simulink library "lib_wheel_nodiv"  (Simulink 7.7)
settings: Solver=ode45  SolverMode=SingleTasking  StartTime=0.0  StopTime=10.0  RelTol=1e-3
undefined symbols (not defined in the file): Fc_table_x, Fc_table_y, I, R, T_veh, use_division, w0, w_max
settings Model: Creator=yt59680  LastModifiedBy=lfeng

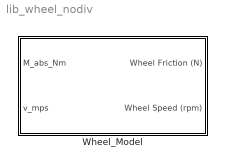
== system lib_wheel_nodiv ==
  Wheel_Model : Subsystem  TreatAsAtomicUnit=on

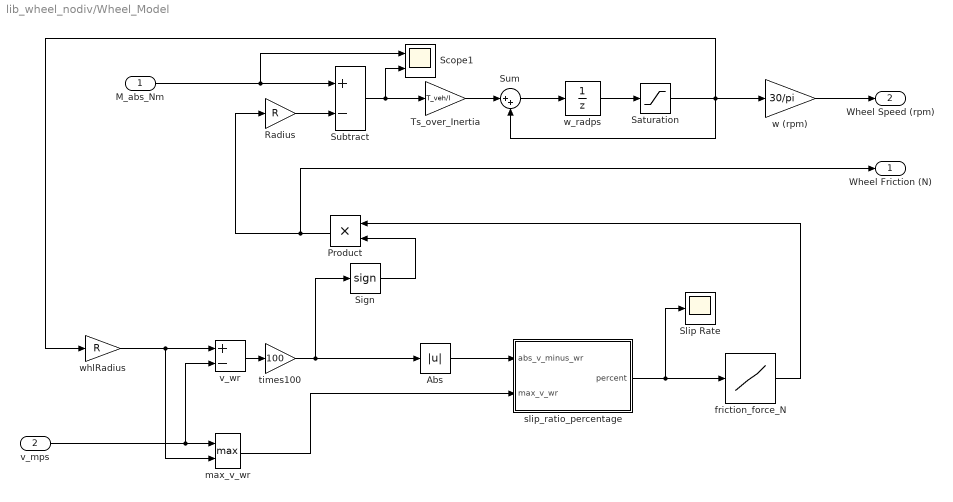
== system lib_wheel_nodiv/Wheel_Model ==
  M_abs_Nm : Inport
  v_mps : Inport  Port=2
  Abs : Abs
  Product : Product  RndMeth=Zero
  Radius : Gain  Gain=R
  Saturation : Saturate  UpperLimit=w_max  LowerLimit=0
  Scope1 : Scope  NumInputPorts=2
      settings: YMin=-5~-5  YMax=5~5  SaveName=ScopeData7
  Sign : Signum
  Slip Rate : Scope
      settings: SaveName=ScopeData8
  Subtract : Sum  Inputs=+-
  Sum : Sum  Inputs=|++
  Ts_over_Inertia : Gain  Gain=T_veh/I
  friction_force_N : Lookup  InputValues=Fc_table_x  Table=Fc_table_y  LookUpMeth=Interpolation-Use End Values  OutMin=0  OutMax=inf  OutDataTypeStr=Inherit: Inherit via back propagation
  max_v_wr : MinMax  Function=max  Inputs=2
  slip_ratio_percentage : Subsystem
  times100 : Gain  Gain=100
  v_wr : Sum  Inputs=+-
  w (rpm) : Gain  Gain=30/pi  OutMin=0  OutMax=w_max*30/pi
  w_radps : UnitDelay  X0=w0  SampleTime=-1
  whlRadius : Gain  Gain=R  OutMin=0  OutMax=w_max/2
  Wheel Friction (N) : Outport
  Wheel Speed (rpm) : Outport  Port=2
  wires:
  times100/1 -> Abs/1, Sign/1
  Saturation/1 -> Sum/2, whlRadius/1, w (rpm)/1
  Sum/1 -> w_radps/1
  friction_force_N/1 -> Product/1
  slip_ratio_percentage/1(percent) -> Slip Rate/1, friction_force_N/1
  whlRadius/1 -> max_v_wr/2, v_wr/1
  Abs/1 -> slip_ratio_percentage/1(abs_v_minus_wr)
  v_wr/1 -> times100/1
  Product/1 -> Wheel Friction (N)/1, Radius/1
  max_v_wr/1 -> slip_ratio_percentage/2(max_v_wr)
  Sign/1 -> Product/2
  Radius/1 -> Subtract/2
  Subtract/1 -> Scope1/2, Ts_over_Inertia/1
  Ts_over_Inertia/1 -> Sum/1
  w_radps/1 -> Saturation/1
  w (rpm)/1 -> Wheel Speed (rpm)/1
  v_mps/1 -> v_wr/2, max_v_wr/1
  M_abs_Nm/1 -> Scope1/1, Subtract/1

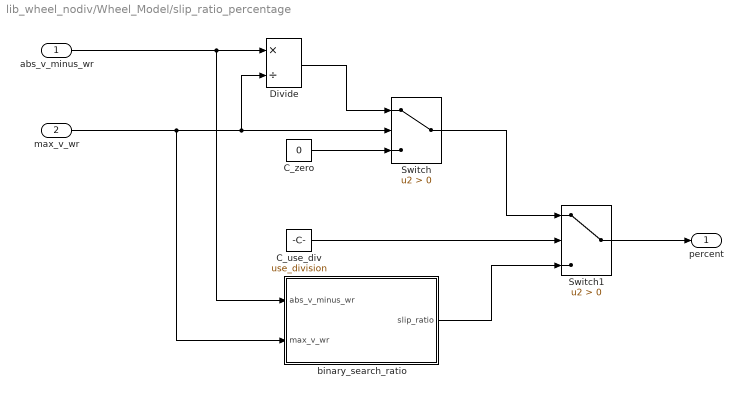
== system lib_wheel_nodiv/Wheel_Model/slip_ratio_percentage ==
  abs_v_minus_wr : Inport
  max_v_wr : Inport  Port=2
  C_use_div : Constant  Value=use_division  SampleTime=-1
  C_zero : Constant  Value=0  SampleTime=-1
  Divide : Product  Inputs=*/
  Switch : Switch  Criteria=u2 > Threshold
  Switch1 : Switch  Criteria=u2 > Threshold
  binary_search_ratio : Stateflow chart  TreatAsAtomicUnit=on
  percent : Outport
  wires:
  binary_search_ratio/1(slip_ratio) -> Switch1/3
  C_use_div/1 -> Switch1/2
  Switch1/1 -> percent/1
  Switch/1 -> Switch1/1
  C_zero/1 -> Switch/3
  Divide/1 -> Switch/1
  abs_v_minus_wr/1 -> binary_search_ratio/1(abs_v_minus_wr), Divide/1
  max_v_wr/1 -> binary_search_ratio/2(max_v_wr), Divide/2, Switch/2

== stateflow chart Wheel_Model/slip_ratio_percentage/binary_search_ratio ==
  (default) -> (junction 3) : /* check boundary conditions */
  (junction 3) -> (junction 5) [order 2]
  (junction 3) -> (junction 6) [order 1] : [abs_v_minus_wr == 0 || max_v_wr == 0]
  (junction 6) -> (junction 7) : {slip_ratio = 0;}
  (junction 5) -> (junction 8) [order 1] : [abs_v_minus_wr >= 100*max_v_wr]
  (junction 8) -> (junction 9) : {slip_ratio = 100;}
  (junction 5) -> (junction 11) [order 2] : {idx_min = 0;
      | idx_max = 99;} /* start binary search */
  (junction 11) -> (junction 10) [order 2] : [idx_max > idx_min]
  (junction 11) -> (junction 9) [order 3] : {slip_ratio = 20;}
      | /* if idx_max < idx_min, return 20%. The case should never happen */
  (junction 7) -> (junction 4) : /* terminate the flow */
  (junction 10) -> (junction 13) : {idx_mid = (idx_min + idx_max)/2;}
      | /* the middle index */
  (junction 13) -> (junction 14) [order 1] : [abs_v_minus_wr < idx_mid * max_v_wr]
      | /* if slip ratio is smaller than idx_mid */
  (junction 14) -> (junction 15) : {idx_max = idx_mid - 1;}
      | /* choose lower part */
  (junction 13) -> (junction 16) [order 2]
  (junction 16) -> (junction 17) [order 1] : [abs_v_minus_wr > (idx_mid + 1)*max_v_wr]
      | /* if slip ratio is larger than idx_mid + 1 */
  (junction 17) -> (junction 15) : {idx_min = idx_mid +1;}
      | /* choose upper part */
  (junction 16) -> (junction 18) [order 2]
  (junction 15) -> (junction 11) : /* go back for iterative search */
  (junction 18) -> (junction 19) [order 1] : [abs_v_minus_wr - idx_mid * max_v_wr <= (idx_mid + 1)*max_v_wr - abs_v_minus_wr]
      | /* if slip ratio is closer to idx_mid than idx_mid + 1 */
  (junction 19) -> (junction 4) : {slip_ratio = idx_mid;}
  (junction 18) -> (junction 12) [order 2] : {slip_ratio = idx_mid + 1;}
  (junction 4) -> (junction 12) : /* terminate the flow */
  (junction 9) -> (junction 7)
  (junction 11) -> (junction 20) [order 1] : [idx_max == idx_min]
      | /* decide if idx_min is idx_max
      | or idx_max + 1 */
  (junction 20) -> (junction 18) : {idx_mid = idx_max;}
  data: abs_v_minus_wr input double; max_v_wr input double; slip_ratio output double [0..100] =0; idx_mid local uint8 size=1 [0..99] =0; idx_min local uint8 size=1 [0..99] =0; idx_max local uint8 size=1 [0..99] =0
